simulink model "denoise_simulink"  (R2019b)
settings: Solver=FixedStepDiscrete  StartTime=0.0  StopTime=39922  RelTol=1e-3
libraries: simulink x2
settings Model: PauseTimes=39000  Creator=meiqiu  LastModifiedBy=Sajib
settings DataIOCC: LoggingToFile=on
settings OptimizationCC: DefaultParameterBehavior=Inlined  UseDivisionForNetSlopeComputation=on  GainParamInheritBuiltInType=on  UseFloatMulNetSlope=on  InlineInvariantSignals=on  PassReuseOutputArgsAs=Individual arguments  ZeroExternalMemoryAtStartup=off  ZeroInternalMemoryAtStartup=off  NoFixptDivByZeroProtection=on  EfficientFloat2IntCast=on  LifeSpan=1  OptimizeBlockOrder=speed  DifferentSizesBufferReuse=on  EfficientTunableParamExpr=on
settings DebuggingCC: ParameterTunabilityLossMsg=error
settings HardwareCC: ProdLongLongMode=on
settings SFSimCC: MATLABDynamicMemAlloc=off  CustomCodeUndefinedFunction=UseInterfaceOnly
settings RTWCC: SystemTargetFile=ert.tlc  TemplateMakefile=ert_default_tmf  GenerateReport=on  IncludeHyperlinkInReport=on  LaunchReport=on  GenerateTraceInfo=on  GenerateTraceReport=on  GenerateTraceReportSl=on  GenerateTraceReportSf=on  GenerateTraceReportEml=on  GenerateCodeMetricsReport=on
settings CodeAppCC: ForceParamTrailComments=on  IgnoreCustomStorageClasses=off  OperatorAnnotations=on  SimulinkDataObjDesc=on  SFDataObjDesc=on  CustomSymbolStrGlobalVar=rt$N$M  CustomSymbolStrType=$N$M  CustomSymbolStrFcn=$N$M$F  CustomSymbolStrMacro=$N$M  InsertBlockDesc=on
settings ERTTargetCC: TargetLangStandard=C99 (ISO)  GenerateSampleERTMain=on  IncludeMdlTerminateFcn=off  CombineSignalStateStructs=on  SuppressErrorStatus=on  SupportComplex=off  InlinedParameterPlacement=NonHierarchical  ERTCustomFileTemplate=example_file_process.tlc  ERTFilePackagingFormat=CompactWithDataFile

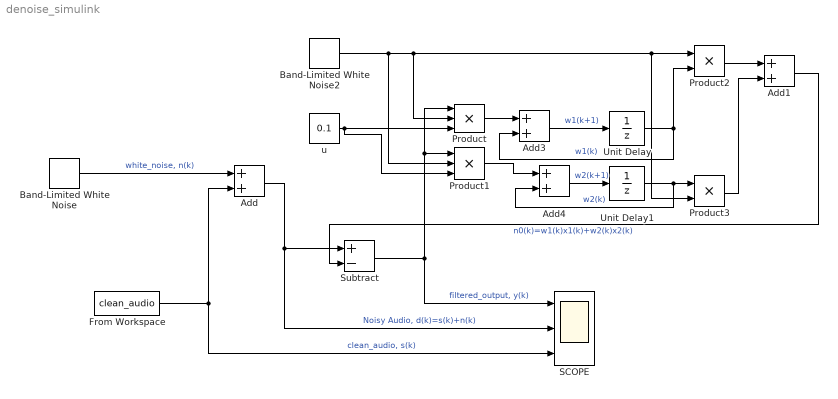
== system denoise_simulink ==
  Add{,1,3..4} (4 alike) : Sum
  Band-Limited White Noise : simulink/Sources/Band-Limited White Noise  Cov=[0.05]  Ts=1  seed=[23341]
  Band-Limited White Noise2 : simulink/Sources/Band-Limited White Noise  Cov=[0.05]  Ts=1  seed=[23341]
  From Workspace : FromWorkspace  VariableName=clean_audio  SampleTime=1  Interpolate=off  OutputAfterFinalValue=Setting to zero
  Product : Product  Inputs=3
  Product1 : Product  Inputs=3
  Product2 : Product
  Product3 : Product
  SCOPE : Scope  NumInputPorts=3
  Subtract : Sum  Inputs=+-
  Unit Delay : UnitDelay  SampleTime=-1  HasFrameUpgradeWarning=on
  Unit Delay1 : UnitDelay  SampleTime=-1  HasFrameUpgradeWarning=on
  u : Constant  Value=0.1
  wires:
  Add4/1 -> Unit Delay1/1  "w2(k+1)"
  Add1/1 -> Subtract/2  "n0(k)=w1(k)x1(k)+w2(k)x2(k)"
  Subtract/1 -> Product1/1, Product/1, SCOPE/1  "filtered_output, y(k)"
  Product3/1 -> Add1/2
  Product/1 -> Add3/1
  Add3/1 -> Unit Delay/1  "w1(k+1)"
  Product1/1 -> Add4/1
  Band-Limited White Noise/1 -> Add/1  "white_noise, n(k)"
  Product2/1 -> Add1/1
  u/1 -> Product1/3, Product/3
  Unit Delay1/1 -> Product3/1, Add4/2  "w2(k)"
  Unit Delay/1 -> Product2/2, Add3/2  "w1(k)"
  Band-Limited White Noise2/1 -> Product3/2, Product2/1, Product/2, Product1/2
  Add/1 -> Subtract/1, SCOPE/2  "Noisy Audio, d(k)=s(k)+n(k)"
  From Workspace/1 -> SCOPE/3, Add/2  "clean_audio, s(k)"
